simulink model "Simulacao_Discreta"  (R2013b)
settings: Solver=ode45  StartTime=0.0  StopTime=5  RelTol=1e-3
undefined symbols (not defined in the file or in its folder): A, B, C, D, dt, k1, k2, k3, PI
settings Model: Creator=Eduardo  LastModifiedBy=Eduardo

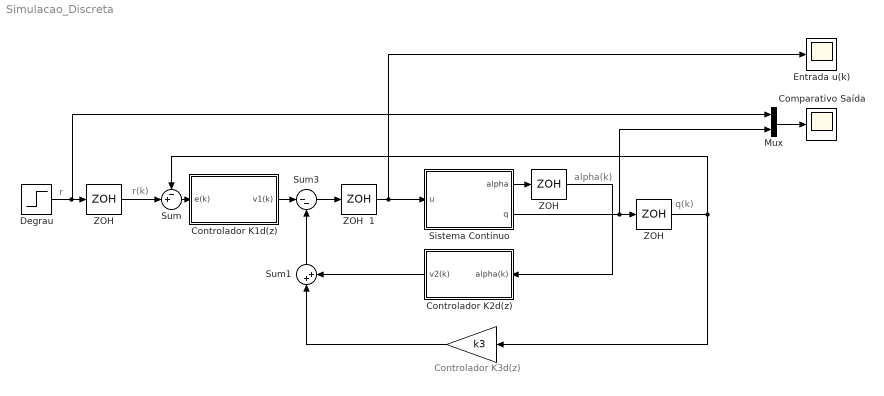
== system Simulacao_Discreta ==
  note: Controlador K3d(z)
  note: alpha(k)
  note: q(k)
  note: r(k)
  note: r
  "    " : Gain  Gain=k3
  Comparativo Saída : Scope
  Controlador K1d(z) : Subsystem
  Controlador K2d(z) : Subsystem
  Degrau : Step  Time=0  SampleTime=0
  Entrada u(k) : Scope
  Mux : Mux  Inputs=2
  "Sistema Contínuo " : Subsystem
  Sum : Sum  Inputs=-+|
  Sum1 : Sum  Inputs=|++
  Sum3 : Sum  Inputs=|--
  ZOH : ZeroOrderHold  SampleTime=dt
  "ZOH " : ZeroOrderHold  SampleTime=dt
  "ZOH  " : ZeroOrderHold  SampleTime=dt
  ZOH  1 : ZeroOrderHold  SampleTime=dt
  wires:
  "Sistema Contínuo "/1(alpha) -> ZOH/1
  Degrau/1 -> "ZOH "/1, Mux/1
  "ZOH "/1 -> Sum/2
  "Sistema Contínuo "/2(q) -> Mux/2, "ZOH  "/1
  "ZOH  "/1 -> "    "/1, Sum/1
  Sum/1 -> Controlador K1d(z)/1(e(k))
  ZOH/1 -> Controlador K2d(z)/1(alpha(k))
  Sum3/1 -> ZOH  1/1
  Mux/1 -> Comparativo Saída/1
  Controlador K2d(z)/1(v2(k)) -> Sum1/2
  Controlador K1d(z)/1(v1(k)) -> Sum3/1
  Sum1/1 -> Sum3/2
  "    "/1 -> Sum1/1
  ZOH  1/1 -> Entrada u(k)/1, "Sistema Contínuo "/1(u)

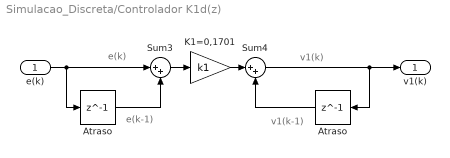
== system Simulacao_Discreta/Controlador K1d(z) ==
  note: v1(k-1)
  note: v1(k)
  note: e(k-1)
  note: e(k)
  e(k) : Inport
  Atraso : Delay  DelayLength=1
  "Atraso " : Delay  DelayLength=1
  K1=0,1701 : Gain  Gain=k1
  Sum3 : Sum  Inputs=|++
  Sum4 : Sum  Inputs=|++
  v1(k) : Outport
  wires:
  Atraso/1 -> Sum3/2
  e(k)/1 -> Sum3/1, Atraso/1
  Sum3/1 -> K1=0,1701/1
  "Atraso "/1 -> Sum4/2
  Sum4/1 -> v1(k)/1, "Atraso "/1
  K1=0,1701/1 -> Sum4/1

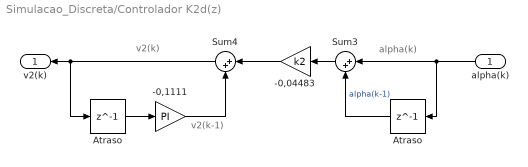
== system Simulacao_Discreta/Controlador K2d(z) ==
  note: v2(k)
  note: alpha(k)
  note: v2(k-1)
  alpha(k) : Inport
  -0,04483 : Gain  Gain=k2
  -0,1111 : Gain  Gain=PI
  Atraso : Delay  DelayLength=1
  "Atraso " : Delay  DelayLength=1
  Sum3 : Sum  Inputs=|++
  Sum4 : Sum  Inputs=|++
  v2(k) : Outport
  wires:
  "Atraso "/1 -> Sum3/2  "alpha(k-1)"
  alpha(k)/1 -> "Atraso "/1, Sum3/1
  Sum4/1 -> Atraso/1, v2(k)/1
  Sum3/1 -> -0,04483/1
  Atraso/1 -> -0,1111/1
  -0,04483/1 -> Sum4/1
  -0,1111/1 -> Sum4/2

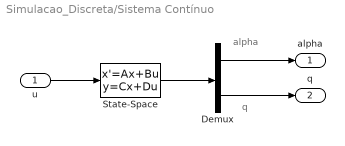
== system Simulacao_Discreta/Sistema Contínuo  ==
  note: alpha
  note: q
  u : Inport
  Demux : Demux  Outputs=2
  State-Space : StateSpace  A=A  B=B  C=C  D=D  X0=0
  alpha : Outport
  q : Outport  Port=2
  wires:
  State-Space/1 -> Demux/1
  u/1 -> State-Space/1
  Demux/2 -> q/1
  Demux/1 -> alpha/1
